simulink model "BUP_FOR_GUI"  (R2018a)
settings: Solver=ode3  StartTime=0.0  StopTime=1000  FixedStep=1  MinStep=1e-8  RelTol=1e-8
undefined symbols (not defined in the file or in its folder): DiscIntNeverNeededParam
libraries: BupSimulinkLibraries x22, simulink_extras x11, SignalEditorBlockLib x2
(part 2 of 2)

== stateflow chart BUP_FOR_GUI/Easy_reg/TaskController ==
  state Timer [parallel]
    entry:
    time = 0;
    during:
    time = time + 1;
    if BimSupply.timeout > 0
    BimSupply.timeout = BimSupply.timeout - 1;
    end
    settings: executionOrder=1
  state Control [parallel]
    % Основной цикл задач
    settings: executionOrder=2
    state Init % Производим планирование путевых точек для сброса высоты
      entry:
      TargetPoint = TDPoint;
      [Flight.Angle.Point1, Flight.Angle.Point2] = AngleManCreator(ActualPoint, TDPoint, AngleManevr);
      [Flight.Box.LUPoint, Flight.Box.LDPoint, Flight.Box.RUPoint, Flight.Box.RDPoint] = BOXCreator(TDPoint, BoxSize);
    state TDP_Only % Режим прицеливания на TDP
      %entry:
      TargetPoint = TDPoint;
    state Flight % Режим полета по точкам
      (history)
      state Angle % Режим углового манёвра
        entry:
        TargetPoint = EntryAngleMan (Point1, Point2, ActualPoint, Course);
      state Box
        % LU - Нацеливание на верхний левый угол "коробки"
        % LD - Нацеливание на нижний левый угол "коробки"
        % RD - Нацеливание на нижний правый угол "коробки"
        % RU - Нацеливание на верхний правый угол "коробки"
        (history)
        state Init
          BoxEntry = VerticeSelect(ActualPoint, LUPoint, LDPoint, RUPoint, RDPoint);
        state RU
          entry:
          TargetPoint = RUPoint;
        state LU
          entry:
          TargetPoint = LUPoint;
        state LD
          entry:
          TargetPoint = LDPoint;
        state RD
          entry:
          TargetPoint = RDPoint;
        (default) -> Init
        Init -> (junction 247)
        (junction 247) -> RU [order 4] : [BoxEntry == 3]
        (junction 247) -> LU [order 1] : [BoxEntry == 1]
        RU -> LU : NextStage
        (junction 247) -> LD [order 3] : [BoxEntry == 2]
        (junction 247) -> RD [order 2] : [BoxEntry == 4]
        LU -> LD : NextStage
        RD -> RU : NextStage
        LD -> RD : NextStage
      state Final
        % Состояние последнего манёвра
        % Цель которого выйти на заданную
        % точку приземления
        entry:
        TargetPoint = TDPoint;
      note: Разрешаем обратные переходы,
          | но с таймаутом, чтобы избежать
          | лишних  переключений
      (default) -> (junction 265)
      (junction 265) -> Box [order 1] : [Mode == 1]
      (junction 265) -> Angle % Режим углового манёвра [order 2] : [Mode == 2]
      Angle % Режим углового манёвра -> Final [order 2] : Final
      Angle % Режим углового манёвра -> Box [order 1] : NextStage
      Box -> Final : Final
      Final -> Box [commented out] : CancelFinal
          | [Timer.timeout == 0]
    (default) -> Init % Производим планирование путевых точек для сброса высоты
    Init % Производим планирование путевых точек для сброса высоты -> (junction 168)
    (junction 168) -> TDP_Only % Режим прицеливания на TDP [order 1] : [Mode == 0]
    (junction 168) -> Flight % Режим полета по точкам [order 2] : [(Mode == 1 || Mode == 2) ]
  note: Данный метод основан на предыдущем механизме прицеливания,
      | однако теперь с помощью Stateflow алгоритм управления будет
      | построен на полете по заданным точкам.
      | Таким образом необходимо организовать планирование полётных точек,
      | и способ их подстановки в мат.модель прицеливания.
  state TargetCourse [parallel]
    %Course2Target = Azimut(TargetPoint, ActualPoint);
    Course2Target = Heading(TargetPoint, ActualPoint, 0);
    settings: executionOrder=3
  state Simulink [group] [commented out]
    % Подсистемы из симулинк блоков
  state Touchdown [parallel]
    %Здесь мы отдельно будем контролировать высоту,
    % для своевременного открытия посадотчных парашютов
    settings: executionOrder=4
    state OFF
      TD_CMD = 0;
    state ON
      TD_CMD = 1;
    (default) -> OFF
    OFF -> (junction 118)
    (junction 124) -> ON : [(ActualPoint(3)-Relief) <= TDPoint(3)]
    (junction 122) -> ON : [ActualPoint(3) <= TDPoint(3)]
    (junction 118) -> (junction 122) [order 1] : [ReliefAvailable == 0]
    (junction 118) -> (junction 124) [order 2] : [ReliefAvailable ==1]
  state EventGenerator [parallel]
    during:
    % Контроль выхода на точку
    if func.CheckFinalMane  == 1;
    Control.Final;
    end
    % Контроль попадания в зону текущей цели
    if CheckArrival(ActualPoint, TargetPoint, ArrivalRadius) == 1;
    Control.NextStage;
    else
    Control.CancelFinal;
    end
    % Контроль попадания в зону точки приземления
    % где на работу БИМов нет ограничений
    if CheckArrival(ActualPoint, TDPoint, 1000) == 1;
    BimSupply.NonBlockingMode;
    end
    % Контроль попадания в зону точки приземления
    % Где управление уже запрещено
    if CheckArrival(ActualPoint, TDPoint, 300) == 1;
    BimSupply.Parking;
    end
    settings: executionOrder=5
  note: Final - Необходимость
      | перенацелиться
      | на точку приземления
      |
      | NextStage - Изменение
      | целевой точки на следу-
      | ющую, согласно алгоритму
      |
      | CancelFinal - На точку
      | приземления выходить
      | рано, высота избыточна
  state func [group]
    % Реализации всех m-функций
  state BimSupply [parallel]
    entry:
    timeout = 0;
    TargetEnable = 1;
    settings: executionOrder=6
    state Enable
      entry:
      TargetEnable = 1;
    state Disable
      entry:
      TargetEnable = 0;
      timeout = 30;
    state NonBlockingControl
      TargetEnable = 1;
    state Shutdown
      TargetEnable = 0;
    (default) -> Enable
    Enable -> Disable [order 2] : [CompletedCorrection  == 1]
    Enable -> NonBlockingControl [order 1] : NonBlockingMode
    Disable -> Enable [order 2] : [timeout == 0]
    Disable -> NonBlockingControl [order 1] : NonBlockingMode
    NonBlockingControl -> Shutdown : Parking
  data: time local uint32 size=1; Point1 local double size=3; Point2 local double size=3; LUPoint local double size=3; LDPoint local double size=3; RUPoint local double size=3; RDPoint local double size=3; BoxEntry local uint8 size=1; Initial_point function_input double size=3; TDP function_input double size=3; AMP1 function_output double size=3; AMP2 function_output double size=3; Angle function_input double size=3; TDP function_input size=3; BLU function_output size=3; BLD function_output size=3; BRU function_output size=3; BRD function_output size=3; BoxStep function_input size=1; InputPoint function_input size=3; OutputPoint function_output size=3; AMP function_input double size=3; BLU function_input double size=3; BLD function_input double size=3; BRU function_input double size=3; BRD function_input double size=3; Vertice function_output uint8 size=1; AM1 function_input double size=3; AM2 function_input double size=3; Position function_input double size=1; point function_output double size=1; TrackingCourse function_input double size=1; Position function_input size=3; Target function_input size=3; y function_output size=1; Now function_input double size=3; To function_input double size=3; status function_output boolean size=1; Radius function_input double size=1; status function_output boolean size=1; To function_input double size=3; From function_input double size=3; y function_output double size=1; timeout local uint32 size=1; Distance output double size=1; T_hor output double size=1; T_ver output double size=1; TDPoint input double size=3; ActualPoint input double size=3; ReliefAvailable input uint8 size=1; Relief input int16 size=1; ReliefOnTDP input int16 size=1; TD_CMD output uint8 size=1; Course input double size=1; BoxSize data_store_memory; ArrivalRadius data_store_memory; AngleManevr data_store_memory; Mode data_store_memory; V_hor input double size=1; V_ver input double size=1; TurnSpeed data_store_memory; Course2TDP input double size=1; TargetEnable output uint8 size=1; CompletedCorrection input boolean size=1; Course2Target output double size=1; TargetPoint local double size=3
  events: Final local FUNCTION_CALL_EVENT; NextStage local FUNCTION_CALL_EVENT; CancelFinal local FUNCTION_CALL_EVENT; Parking local FUNCTION_CALL_EVENT; NonBlockingMode local FUNCTION_CALL_EVENT
  function [AMP1, AMP2] = AngleManCreator(Initial_point, TDP, Angle):
    | %%%%%%%%%%%%%%%%%%%%%%%%%%%%%%%%%%%%%%%%%%%%%%%%%%%%%%%%%%%%%%%%%%%%%%%%%%%
    | % AngleManCreator - Создание точек углового манёвра по обе стороны от ЛЗП
    | %%%%%%%%%%%%%%%%%%%%%%%%%%%%%%%%%%%%%%%%%%%%%%%%%%%%%%%%%%%%%%%%%%%%%%%%%%%
    | function [AMP1, AMP2] = AngleManCreator(Initial_point, TDP, Angle)
    |     %% Расшифровка переменных
    |     % AMP - Координата углового манёвра
    |     %% Это точка углового манёвра расчитанная по равностороннему треугольнику
    |     x1 = Initial_point(2);
    |     y1 = Initial_point(1);
    |     x2 = TDP(2);
    |     y2 = TDP(1);
    |     % Возьмем половину расстояния до точки посадки и повернём этот вектор на
    |     dx = (x2-x1)/2;
    |     dy = (y2-y1)/2;
    |     % Определяем первую точку
    |     x3 = dx*cos(Angle*pi/180) - dy*sin(Angle*pi/180)+x1;
    |     y3 = dx*sin(Angle*pi/180) + dy*cos(Angle*pi/180)+y1;
    |     AMP1 = [y3;x3;0];
    |     % Определяем вторую точку
    |     x4 = dx*cos(-Angle*pi/180) - dy*sin(-Angle*pi/180)+x1;
    |     y4 = dx*sin(-Angle*pi/180) + dy*cos(-Angle*pi/180)+y1;
    |     AMP2 = [y4;x4;0];
    |     %% Проверим выход точек за пределы координат
    |     AMP1 = PositionRangeConverting(AMP1);
    |     AMP2 = PositionRangeConverting(AMP2);
    | end
  function [BLU, BLD, BRU, BRD] = BOXCreator(TDP, BoxStep):
    | %%%%%%%%%%%%%%%%%%%%%%%%%%%%%%%%%%%%%%%%%%%%%%%%%%%%%%%%%%%%%%%%%%%%%%%%%%%
    | % BOXCreator - Создание опорных точек аварийного манёвра "Коробка"
    | %%%%%%%%%%%%%%%%%%%%%%%%%%%%%%%%%%%%%%%%%%%%%%%%%%%%%%%%%%%%%%%%%%%%%%%%%%%
    | function [BLU, BLD, BRU, BRD] = BOXCreator(TDP, BoxStep)
    |     %% Расшифровка переменных
    |     % BLU - Координата верхней левой точки квадрата
    |     % BLD - Координата нижней левой точки квадрата
    |     % BRU - Координата верхней правой точки квадрата
    |     % BRD - Координата нижней правой точки квадрата
    |     %% Расчитываем точки квадрата
    |     BLU=[0; 0; 0]; BLD = [0; 0; 0]; BRU = [0; 0; 0]; BRD=[0; 0; 0];
    |     % Вычисляем шаг в градусах по Широте (однозначно сопоставляются)
    |     LatStep = BoxStep/1000*360/40000;
    |     % Координаты по Широте
    |     BLU(1) = TDP(1) + LatStep;
    |     BLD(1) = TDP(1) - LatStep; 
    |     BRU(1) = TDP(1) + LatStep;
    |     BRD(1) = TDP(1) - LatStep; 
    |     % Вычисляем шаг по Долготе без учета поправки на Широту (долгота зависит от
    |     % широты), а поправку на широту будем делать прямо в выражении
    |     LonStep = BoxStep/1000*360/40000;
    |     % Координаты по Долготе
    |     BLU(2) = TDP(2) - LonStep/cos(pi*BLU(1)/180);
    |     BLD(2) = TDP(2) - LonStep/cos(pi*BLD(1)/180);
    |     BRU(2) = TDP(2) + LonStep/cos(pi*BRU(1)/180);
    |     BRD(2) = TDP(2) + LonStep/cos(pi*BRD(1)/180);
    |     %% Проверим выход точек за пределы координат
    |     BLU = PositionRangeConverting(BLU);
    |     BLD = PositionRangeConverting(BLD);
    |     BRU = PositionRangeConverting(BRU);
    |     BRD = PositionRangeConverting(BRD);
    | end
  function OutputPoint = PositionRangeConverting(InputPoint):
    | %%%%%%%%%%%%%%%%%%%%%%%%%%%%%%%%%%%%%%%%%%%%%%%%%%%%%%%%%%%%%%%%%%%%%%%%%%%
    | % PositionRangeConverting - Проверка корректности сферических координат 
    | %%%%%%%%%%%%%%%%%%%%%%%%%%%%%%%%%%%%%%%%%%%%%%%%%%%%%%%%%%%%%%%%%%%%%%%%%%%
    | function OutputPoint = PositionRangeConverting(InputPoint)
    |     %% Контроль пределов Координат
    |     % InputPoint(1) - Широта
    |     % InputPoint(2) - Долгота
    |     % InputPoint(3) - Высота
    |     OutputPoint = InputPoint;
    |     %% Преобразование Долготы
    |     if OutputPoint(2) > 180
    |         OutputPoint(2) = OutputPoint(2) - 360;
    |     elseif OutputPoint(2) < (-180)
    |         OutputPoint(2) = OutputPoint(2) + 360;
    |     end
    | end
  function Vertice = VerticeSelect(AMP, BLU, BLD, BRU, BRD):
    | %%%%%%%%%%%%%%%%%%%%%%%%%%%%%%%%%%%%%%%%%%%%%%%%%%%%%%%%%%%%%%%%%%%%%%%%%%%
    | %  VerticeSelect - Выбор оптимального входа в манёвр "коробка"
    | %
    | %  AMP - Координаты точки, от которой расчитывается вход
    | %  BLU - Координаты точки левого верхнего угла коробки
    | %  BLD - Координаты точки левого нижнего угла коробки 
    | %  BRU - Координаты точки правого верхнего угла коробки 
    | %  BRD - Координаты точки нижнего верхнего угла коробки
    | %
    | %  Возвращает номер вершины оптимального входа
    | %      1 - BLU, 2 - BLD, 3 - BRU, 4 - BRD
    | %%%%%%%%%%%%%%%%%%%%%%%%%%%%%%%%%%%%%%%%%%%%%%%%%%%%%%%%%%%%%%%%%%%%%%%%%%%
    | function Vertice = VerticeSelect(AMP, BLU, BLD, BRU, BRD)
    |     %% Функция определения точки входа в "посадочной коробке"
    |     D_BLU = DistanceCalculator(AMP,BLU);
    |     D_BLD = DistanceCalculator(AMP,BLD);
    |     D_BRU = DistanceCalculator(AMP,BRU);
    |     D_BRD = DistanceCalculator(AMP,BRD);
    |     %% Соответсвие значения Vertice и вершин коробки
    |     % 1 - Левая верхняя
    |     % 2 - Левая нижняя
    |     % 3 - Правая верхняя
    |     % 4 - Правая нижняя
    |     x = [D_BLU, D_BLD, D_BRU, D_BRD]; 
    |     Vertice = 1;
    |     for i = 1:1:3
    |         if x(i+1) < x(Vertice)
    |             Vertice = i+1;
    |         end
    |     end
    |     Vertice = uint8(Vertice);
    | end
  function point = EntryAngleMan (AM1, AM2, Position, TrackingCourse):
    | %%%%%%%%%%%%%%%%%%%%%%%%%%%%%%%%%%%%%%%%%%%%%%%%%%%%%%%%%%%%%%%%%%%%%%%%%%%
    | % EntryAngleMan - Определение оптимальной точки входа в угловой манёвр
    | % AM1            - Точка углового манёвра 1
    | % AM2            - Точка углового манёвра 2
    | % Position       - Текущие координаты
    | % TrackingCourse - Текущий курс
    | %
    | % Возвращает одну из точек (AM1 или AM2) в зависимости от оптимальности
    | %%%%%%%%%%%%%%%%%%%%%%%%%%%%%%%%%%%%%%%%%%%%%%%%%%%%%%%%%%%%%%%%%%%%%%%%%%%
    | function point = EntryAngleMan (AM1, AM2, Position, TrackingCourse)
    |     %% Определим курс до точек манёвра
    |     Course1 = CourseCalculator(AM1, Position);
    |     Course2 = CourseCalculator(AM2, Position);
    |     %% Найдём разницу с путевым
    |     Course1 = Course1 - TrackingCourse;
    |     Course2 = Course2 - TrackingCourse;
    |     %% Проведем нормирование разницы
    |     if Course1 > pi
    |         Course1 = Course1 - 2*pi;
    |     end
    |     if Course1 < (-pi)
    |         Course1 = Course1 + 2*pi;
    |     end
    |     if Course2 > pi
    |         Course2 = Course2 - 2*pi;
    |     end
    |     if Course2 < (-pi)
    |         Course2 = Course2 + 2*pi;
    |     end
    |     %% Возьмём модуль для сравнения
    |     Course1 = abs(Course1);
    |     Course2 = abs(Course2);
    |     %% Будет выбрана точка до которой поворот меньше
    |     if Course1 < Course2
    |         point = AM1;
    |     else
    |         point = AM2;
    |     end
    | end
  function y = DistanceCalculator (Position, Target):
    | %%%%%%%%%%%%%%%%%%%%%%%%%%%%%%%%%%%%%%%%%%%%%%%%%%%%%%%%%%%%%%%%%%%%%%%%%%%
    | % DistanceCalculator - Вычисление расстрояния от Position до Target 
    | % в метрах по сферическим координатам
    | %%%%%%%%%%%%%%%%%%%%%%%%%%%%%%%%%%%%%%%%%%%%%%%%%%%%%%%%%%%%%%%%%%%%%%%%%%%
    | function y = DistanceCalculator (Position, Target)
    |     %% Вычитаем расстояние (через вектора)
    |     % dif = (TDP - ActualPoint);
    |     % % Вычисляем проекции на оси с переводом в Км.
    |     % distance_lon2x = dif(1)*40000/360*cos(dif(2)*pi/180);
    |     % distance_lat2y = dif(2)*40000/360;
    |     % distance = sqrt(distance_lon2x^2 + distance_lat2y^2);
    |     %% Вычитаем расстояние (через тригонометрию)
    |     la1 = Position(2)*pi/180;
    |     fi1 = Position(1)*pi/180;
    |     la2 = Target(2)*pi/180;
    |     fi2 = Target(1)*pi/180;
    |     d = sin(fi1)*sin(fi2) + cos(fi1)*cos(-fi2)*cos(la2-la1);
    |     % 6371 км средний радиус земли
    |     y = acos(d)*6371e3;
    | end
  function status = CheckArrival (Now, To, Radius):
    | %%%%%%%%%%%%%%%%%%%%%%%%%%%%%%%%%%%%%%%%%%%%%%%%%%%%%%%%%%%%%%%%%%%%%%%%%%%
    | % CheckArrival - Проверка прибытия в точку с координатами "To"
    | % Now    - Текущие координаты
    | % To     - Координаты точки приземления
    | % Radius - Радиус зоны попадания, м
    | %%%%%%%%%%%%%%%%%%%%%%%%%%%%%%%%%%%%%%%%%%%%%%%%%%%%%%%%%%%%%%%%%%%%%%%%%%%
    | function status = CheckArrival (Now, To, Radius)
    |     %% Вычитаем коррдинаты и берем модуль
    |     %dif = (To - Now);
    |     %distance = sqrt(dif(1)^2 + dif(2)^2);
    |     %% Вычисляем расстояние с помощью DistanceCalculator
    |     distance = DistanceCalculator (Now, To);
    |     %% Попаданием будем считать радиус 
    |     if distance < Radius
    |         status = 1;
    |     else
    |         status = 0;
    |     end
    | end
  function status = CheckFinalMane:
    | %%%%%%%%%%%%%%%%%%%%%%%%%%%%%%%%%%%%%%%%%%%%%%%%%%%%%%%%%%%%%%%%%%%%%%%%%%%
    | % CheckFinalMane - Проверка необходимости перехода к финальному манёвру
    | %
    | % Использует глобальные переменные:
    | %    ActualPoint - Текущие координаты
    | %    TDPoint     - Координаты точки приземления
    | %    V_hor       - Горизонтальная скорость полета (м/с)
    | %    V_ver       - Скорость снижения (м/c)
    | %    Course      - Путевой курс
    | %    Course2TDP  - Курс (азимут) до точки приземления
    | %    ReliefOnTDP - Высота рельефа над точкой приземления
    | %
    | %%%%%%%%%%%%%%%%%%%%%%%%%%%%%%%%%%%%%%%%%%%%%%%%%%%%%%%%%%%%%%%%%%%%%%%%%%%
    | function status = CheckFinalMane ()
    |     %% Вычислим расстояние с помощью функции DistanceCalculator()
    |     Distance = DistanceCalculator(ActualPoint, TDPoint);
    |     %% Вычисляем время необходимое для преодоления расстояния до TDP и до посадки
    |     T_hor = Distance/V_hor;
    |     T_ver = (ActualPoint(3) - (TDPoint(3) + double(ReliefOnTDP)))/V_ver;
    |     %% Определяем поправку по времени необходимому на разворот
    |     % Угол разворота
    |     angle = abs(Course2TDP-Course) * 180 / pi;
    |     if angle > 180
    |         angle = angle - 180;
    |     end
    | 
    |     % Вычисляем поправку как линейную функцию: 
    |     T_hor_popr = angle / TurnSpeed;
    | 
    |     % Вычисляем поправку по параболе
    |     %T_hor_popr = 0.003*angle^2 + 0.008*angle;
    | 
    |     T_hor = T_hor + T_hor_popr;
    |     %% Возвращаем сигнал о необходимости перейти на финальный маневр
    |     if T_hor > T_ver
    |         status = 1;
    |     else
    |         status = 0;
    |     end
    | end
  function y = CourseCalculator(To, From):
    | %%%%%%%%%%%%%%%%%%%%%%%%%%%%%%%%%%%%%%%%%%%%%%%%%%%%%%%%%%%%%%%%%%%%%%%%%%%
    | % CourseCalculator - Вычисление азимута от точки FROM до точки TO
    | %%%%%%%%%%%%%%%%%%%%%%%%%%%%%%%%%%%%%%%%%%%%%%%%%%%%%%%%%%%%%%%%%%%%%%%%%%%
    | function y = CourseCalculator(To, From)
    | %% Высчитаем, как изменились координаты
    | un = To - From;
    | d_lat = un(1);
    | d_lon = un(2);
    | %% Условие для определения кратчайшего пути с учетом переходов между
    | % меридианами 0 и 180 по долготе
    | if d_lon > 180
    |     d_lon = d_lon - 360;
    | elseif d_lon < (-180)
    |         d_lon = d_lon +360;
    | end
    | %% Расчет курса
    | un_pow1 = d_lat*d_lat;
    | un_pow2 = d_lon*d_lon;
    | if (un_pow1 < 1e-16) && (un_pow2 < 1e-16)
    |     y = 0;
    | else
    |     x = acos( d_lon / (sqrt(un_pow2 + un_pow1)));
    |     y = acos( d_lat / (sqrt(un_pow2 + un_pow1)));
    |     if x > 1.5708
    |         y = 6.28319 - y;
    |     end
    | end
